simulink model "Actuator_Primitives"  (R2012b)
settings: Solver=FixedStepDiscrete  StartTime=0.0  StopTime=10.0  FixedStep=0.1  RelTol=1e-3
settings Model: Creator=Kerianne  LastModifiedBy=Kerianne
settings DataIOCC: SaveFormat=Structure
settings OptimizationCC: InlineParams=on

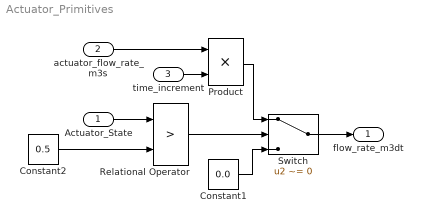
== system Actuator_Primitives ==
  Actuator_State : Inport
  actuator_flow_rate_m3s : Inport  Port=2
  time_increment : Inport  Port=3
  Constant1 : Constant  Value=0.0
  Constant2 : Constant  Value=0.5
  Product : Product
  Relational Operator : RelationalOperator  Operator=>  OutDataTypeStr=boolean
  Switch : Switch  Criteria=u2 ~= 0
  flow_rate_m3dt : Outport
  wires:
  time_increment/1 -> Product/2
  Product/1 -> Switch/1
  Switch/1 -> flow_rate_m3dt/1
  actuator_flow_rate_m3s/1 -> Product/1
  Constant2/1 -> Relational Operator/2
  Constant1/1 -> Switch/3
  Actuator_State/1 -> Relational Operator/1
  Relational Operator/1 -> Switch/2
